simulink model "dcmotor_lab1"  (R2023b)
settings: Solver=VariableStepAuto  StartTime=0.0  StopTime=100  RelTol=1e-3
undefined symbols (not defined in the file): Kb, Kt, La, Ra
libraries: simulink_extras x18
settings Model: Creator=kuotz  LastModifiedBy=kuotz

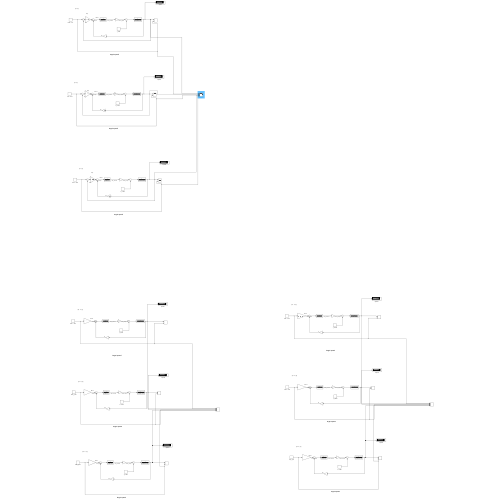
[thumbnail: Simulink's stored preview of the top-level diagram]
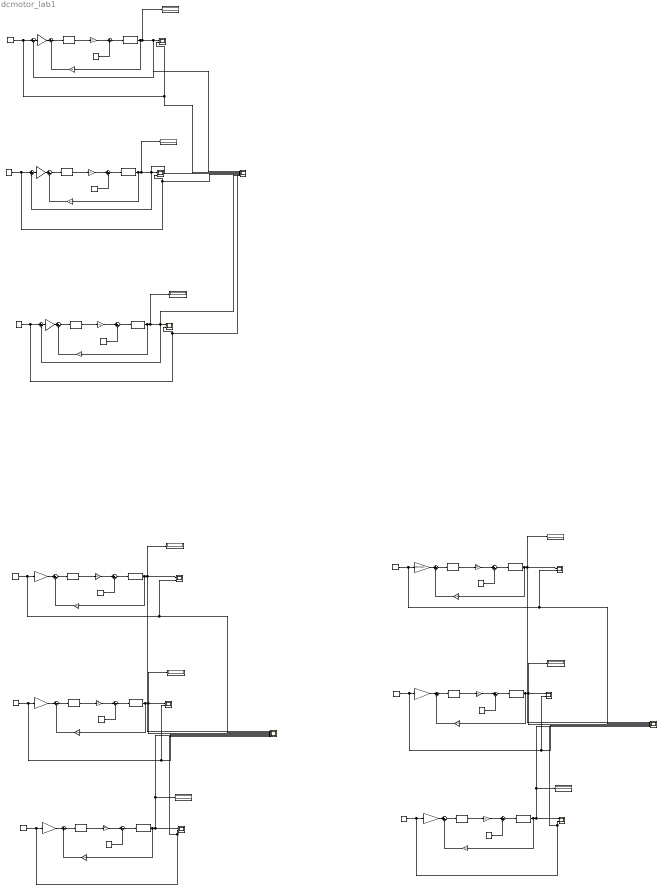
== system dcmotor_lab1 ==
  note: Kvp
  note: target speed
  note: 第c小題
  note: error
  note: e
  note: Ea=vt
  note: target speed
  note: 第a、b小題
  note: Ea=vt
  note: target speed
  note: 第a、b小題
  note: Ea=vt
  note: target speed
  note: Ea=vt
  note: 第a、b小題
  note: 第c小題
  note: target speed
  note: e
  note: Ea=vt
  note: error
  note: 第c小題
  note: target speed
  note: e
  note: Ea=vt
  note: error
  note: Kvp
  note: Kvp
  note: Ea=vt
  note: target speed
  note: target speed
  note: Ea=vt
  note: 第a、b小題
  note: 第a、b小題
  note: target speed
  note: Ea=vt
  note: 第a、b小題
  Gain{,3,6,9,12,15,20,23,26} (9 alike) : Gain  Gain=Kt
  Gain{1,4,7,10,13,16,18,21,24} (9 alike) : Gain  Gain=Kb
  Gain{5,8,11,22} (4 alike) : Gain  Gain=250/3000
  Gain14 : Gain  Gain=47.7552
  Gain17 : Gain  Gain=47.7558
  Gain19 : Gain  Gain=251.4/3000
  Gain2 : Gain  Gain=47.7548
  Gain25 : Gain  Gain=252.9/3000
  Scope{,2..6,9..11} (9 alike) : Scope  NumInputPorts=2
  Scope1 : Scope  NumInputPorts=6
  Scope7 : Scope  NumInputPorts=6
  Scope8 : Scope  NumInputPorts=6
  Speed{,1..8} (9 alike) : Display
  Sum{,1..20} (21 alike) : Sum  Inputs=|+-
  T_Load{,4..8} (6 alike) : Constant  Value=1.2
  T_Load1 : Constant  Value=0
  T_Load2 : Constant  Value=0
  T_Load3 : Constant  Value=0
  Transfer Fcn (with initial states){,2,4,6,8,10,12,14,16} (9 alike) : simulink_extras/Additional Linear/Transfer Fcn (with initial states)  N=[1]  D="[La  Ra]"  X0=.5
  Transfer Fcn (with initial states){1,3,5,7,9,11,13,15,17} (9 alike) : simulink_extras/Additional Linear/Transfer Fcn (with initial states)  N=[1]  D="[0.03760  0.001]"  X0=.5
  theta_r_dot : Constant  Value=1000
  theta_r_dot1 : Constant  Value=1000
  theta_r_dot2 : Constant  Value=1500
  theta_r_dot3 : Constant  Value=3000
  theta_r_dot4 : Constant  Value=1500
  theta_r_dot5 : Constant  Value=3000
  theta_r_dot6 : Constant  Value=1000
  theta_r_dot7 : Constant  Value=1500
  theta_r_dot8 : Constant  Value=3000
  wires:
  Sum/1 -> Transfer Fcn (with initial states)/1
  Transfer Fcn (with initial states)/1 -> Gain/1  "Arm_Current"
  Gain/1 -> Sum1/1  "motor_torque"
  Sum1/1 -> Transfer Fcn (with initial states)1/1
  T_Load/1 -> Sum1/2
  Gain1/1 -> Sum/2  "Eb"
  Transfer Fcn (with initial states)1/1 -> Scope7/1, Sum2/2, Scope/1, Speed/1, Gain1/1
  Sum2/1 -> Gain2/1
  Gain2/1 -> Sum/1  "motor_torque"
  theta_r_dot/1 -> Scope7/2, Scope/2, Sum2/1
  theta_r_dot1/1 -> Scope2/2, Scope1/2, Gain5/1
  Gain4/1 -> Sum3/2  "Eb"
  T_Load1/1 -> Sum4/2
  Sum4/1 -> Transfer Fcn (with initial states)3/1
  Gain3/1 -> Sum4/1  "motor_torque"
  Transfer Fcn (with initial states)2/1 -> Gain3/1  "Arm_Current"
  Sum3/1 -> Transfer Fcn (with initial states)2/1
  Gain5/1 -> Sum3/1  "motor_torque"
  Gain8/1 -> Sum5/1  "motor_torque"
  Sum5/1 -> Transfer Fcn (with initial states)4/1
  Transfer Fcn (with initial states)4/1 -> Gain6/1  "Arm_Current"
  Gain6/1 -> Sum6/1  "motor_torque"
  Sum6/1 -> Transfer Fcn (with initial states)5/1
  T_Load2/1 -> Sum6/2
  Gain7/1 -> Sum5/2  "Eb"
  Transfer Fcn (with initial states)5/1 -> Scope3/1, Scope1/3, Speed2/1, Gain7/1
  Gain11/1 -> Sum7/1  "motor_torque"
  Transfer Fcn (with initial states)7/1 -> Scope4/1, Scope1/5, Speed3/1, Gain10/1
  Sum8/1 -> Transfer Fcn (with initial states)7/1
  Gain10/1 -> Sum7/2  "Eb"
  theta_r_dot3/1 -> Scope4/2, Scope1/6, Gain11/1
  Sum7/1 -> Transfer Fcn (with initial states)6/1
  T_Load3/1 -> Sum8/2
  Transfer Fcn (with initial states)6/1 -> Gain9/1  "Arm_Current"
  Gain9/1 -> Sum8/1  "motor_torque"
  Transfer Fcn (with initial states)3/1 -> Gain4/1, Scope1/1, Scope2/1, Speed1/1
  theta_r_dot2/1 -> Scope3/2, Scope1/4, Gain8/1
  theta_r_dot4/1 -> Scope7/4, Scope5/2, Sum11/1
  Sum11/1 -> Gain14/1
  Gain14/1 -> Sum9/1  "motor_torque"
  Gain13/1 -> Sum9/2  "Eb"
  Transfer Fcn (with initial states)8/1 -> Gain12/1  "Arm_Current"
  T_Load4/1 -> Sum10/2
  Sum10/1 -> Transfer Fcn (with initial states)9/1
  Transfer Fcn (with initial states)9/1 -> Scope7/3, Sum11/2, Scope5/1, Speed4/1, Gain13/1
  Sum9/1 -> Transfer Fcn (with initial states)8/1
  Gain12/1 -> Sum10/1  "motor_torque"
  theta_r_dot5/1 -> Scope7/6, Scope6/2, Sum14/1
  Sum14/1 -> Gain17/1
  Gain17/1 -> Sum12/1  "motor_torque"
  Gain16/1 -> Sum12/2  "Eb"
  Transfer Fcn (with initial states)10/1 -> Gain15/1  "Arm_Current"
  T_Load5/1 -> Sum13/2
  Sum13/1 -> Transfer Fcn (with initial states)11/1
  Transfer Fcn (with initial states)11/1 -> Scope7/5, Sum14/2, Scope6/1, Speed5/1, Gain16/1
  Sum12/1 -> Transfer Fcn (with initial states)10/1
  Gain15/1 -> Sum13/1  "motor_torque"
  Gain19/1 -> Sum19/1  "motor_torque"
  Sum20/1 -> Transfer Fcn (with initial states)17/1
  Transfer Fcn (with initial states)17/1 -> Scope11/1, Scope8/5, Speed8/1, Gain18/1
  Gain26/1 -> Sum20/1  "motor_torque"
  Transfer Fcn (with initial states)16/1 -> Gain26/1  "Arm_Current"
  Sum19/1 -> Transfer Fcn (with initial states)16/1
  theta_r_dot8/1 -> Scope11/2, Scope8/6, Gain19/1
  Transfer Fcn (with initial states)12/1 -> Gain20/1  "Arm_Current"
  Sum16/1 -> Transfer Fcn (with initial states)13/1
  T_Load6/1 -> Sum16/2
  Transfer Fcn (with initial states)13/1 -> Gain21/1, Scope8/1, Scope9/1, Speed6/1
  theta_r_dot6/1 -> Scope9/2, Scope8/2, Gain22/1
  Sum15/1 -> Transfer Fcn (with initial states)12/1
  T_Load8/1 -> Sum20/2
  Gain21/1 -> Sum15/2  "Eb"
  Gain22/1 -> Sum15/1  "motor_torque"
  Gain20/1 -> Sum16/1  "motor_torque"
  Gain25/1 -> Sum17/1  "motor_torque"
  Transfer Fcn (with initial states)15/1 -> Scope10/1, Scope8/3, Speed7/1, Gain24/1
  Sum18/1 -> Transfer Fcn (with initial states)15/1
  Sum17/1 -> Transfer Fcn (with initial states)14/1
  Gain18/1 -> Sum19/2  "Eb"
  T_Load7/1 -> Sum18/2
  Transfer Fcn (with initial states)14/1 -> Gain23/1  "Arm_Current"
  Gain23/1 -> Sum18/1  "motor_torque"
  Gain24/1 -> Sum17/2  "Eb"
  theta_r_dot7/1 -> Scope10/2, Scope8/4, Gain25/1
